simulink model "mpc_cvxgen"  (R2015b)
settings: Solver=VariableStepAuto  StartTime=0.0  StopTime=50  FixedStep=Ts  RelTol=1e-3
InitFcn:
  | mpc_trajectory_data_callback
values from neighbouring files (symbols this model uses):
  Ts = 1    [example_mpc_cycle.m]    (also in init_mpc_test.m = 0.2)
undefined symbols (not defined in the file or in its folder): sCoeffs, sPolyorder, sTimes
undefined symbols (not defined in the file): CVXparameters
settings Model: Creator=Daniel  LastModifiedBy=mgreiff
settings SolverCC: AlgebraicLoopSolver=LineSearch

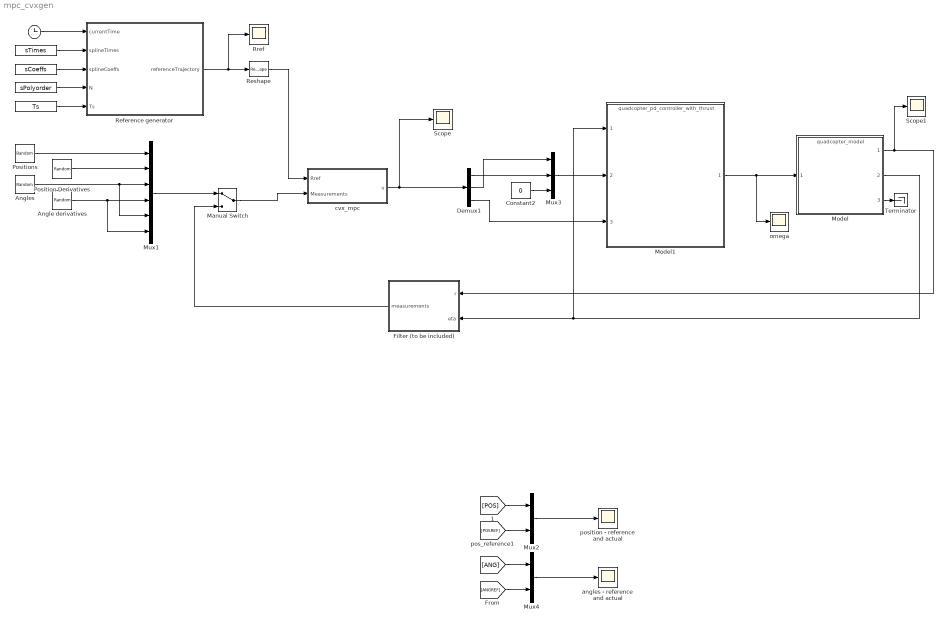
== system mpc_cvxgen ==
  " " : Constant  Value=Ts
  "  " : Constant  Value=sPolyorder
  "   " : Constant  Value=sCoeffs
  "    " : Constant  Value=sTimes
  "      " : Clock
  "  angles - reference and actual" : Scope
  "  position - reference and actual" : Scope
  Angle derivatives : RandomNumber  Variance=0.1  SampleTime=Ts
  Angles : RandomNumber  Variance=0.1  SampleTime=Ts
  Constant2 : Constant  Value=0
  Demux1 : Demux  Outputs=3
  Filter (to be included) : Subsystem
  Manual Switch : ManualSwitch
  Model : ModelReference  ModelNameDialog=quadcopter_model.mdl  SimulationMode=Normal  ModelReferenceVersion=1.114  CopyOfModelName=quadcopter_model.mdl
  Model1 : ModelReference  ModelNameDialog=quadcopter_pd_controller_with_thrust.mdl  SimulationMode=Normal  ModelReferenceVersion=1.70  CopyOfModelName=quadcopter_pd_controller_with_thrust.mdl
  Mux1 : Mux  Inputs=6
  Mux2 : Mux  Inputs=2
  Mux3 : Mux  Inputs=3
  Mux4 : Mux  Inputs=2
  Position Derivatives : RandomNumber  Mean=[0,0,0]  Variance=0.1  SampleTime=Ts
  Positions : RandomNumber  Mean=[0,0,0]  Variance=0.1  SampleTime=Ts
  Reference generator : MATLAB Function  TreatAsAtomicUnit=on
  Reshape : Reshape
  Rref : Scope
  Scope : Scope
  Scope1 : Scope
  Terminator : Terminator
  cvx_mpc : Subsystem  mask{md=CVXparameters}
      mask prompts: md "MPCData"
  "omega " : Scope
  wires:
  Angles/1 -> Mux1/5, Mux1/3
  Angle derivatives/1 -> Mux1/6, Mux1/4
  Positions/1 -> Mux1/1
  Position Derivatives/1 -> Mux1/2
  "      "/1 -> Reference generator/1(currentTime)
  "    "/1 -> Reference generator/2(splineTimes)
  "   "/1 -> Reference generator/3(splineCoeffs)
  "  "/1 -> Reference generator/4(N)
  " "/1 -> Reference generator/5(Ts)
  Reshape/1 -> cvx_mpc/1(Rref)
  Reference generator/1(referenceTrajectory) -> Rref/1, Reshape/1
  Mux1/1 -> Manual Switch/1
  Manual Switch/1 -> cvx_mpc/2(Measurements)
  cvx_mpc/1(u) -> Scope/1, Demux1/1
  Demux1/3 -> Model1/3
  Mux3/1 -> Model1/2
  Constant2/1 -> Mux3/3
  Demux1/2 -> Mux3/1
  Demux1/1 -> Mux3/2
  Model1/1 -> Model/1, "omega "/1
  [POS] -> Mux2/1
  [POSREF] -> Mux2/2
  Mux2/1 -> "  position - reference and actual"/1
  Model/2 -> Filter (to be included)/2(eta), Model1/1
  Filter (to be included)/1(measurements) -> Manual Switch/2
  [ANG] -> Mux4/1
  [ANGREF] -> Mux4/2
  Mux4/1 -> "  angles - reference and actual"/1
  Model/1 -> Scope1/1, Filter (to be included)/1(r)
  Model/3 -> Terminator/1

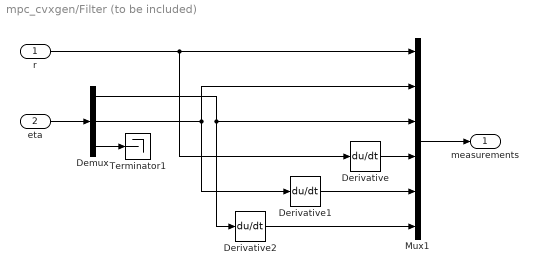
== system mpc_cvxgen/Filter (to be included) ==
  r : Inport
  eta : Inport  Port=2
  Demux : Demux  Outputs=3
  Derivative : Derivative
  Derivative1 : Derivative
  Derivative2 : Derivative
  Mux1 : Mux  Inputs=6
  Terminator1 : Terminator
  measurements : Outport
  wires:
  Demux/1 -> Mux1/3, Derivative2/1
  Derivative/1 -> Mux1/4
  Derivative2/1 -> Mux1/6
  Demux/3 -> Terminator1/1
  Demux/2 -> Mux1/2, Derivative1/1
  Derivative1/1 -> Mux1/5
  r/1 -> Derivative/1, Mux1/1
  eta/1 -> Demux/1
  Mux1/1 -> measurements/1

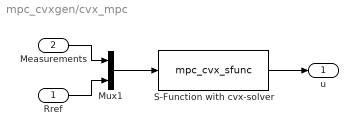
== system mpc_cvxgen/cvx_mpc ==
  Rref : Inport
  Measurements : Inport  Port=2
  Mux1 : Mux  Inputs=2
  S-Function with cvx-solver : S-Function  FunctionName=mpc_cvx_sfunc  Parameters=CVXparameters  SFunctionDeploymentMode=off  EnableBusSupport=off
  u : Outport
  wires:
  Measurements/1 -> Mux1/1
  Rref/1 -> Mux1/2
  S-Function with cvx-solver/1 -> u/1
  Mux1/1 -> S-Function with cvx-solver/1

== matlab function mpc_cvxgen/Reference generator ==
  data: currentTime input; referenceTrajectory output; splineTimes input; splineCoeffs input; N input; Ts input
function referenceTrajectory = fcn(currentTime, splineTimes, splineCoeffs, N, Ts)
%#codegen

predHorizon = 10 + 1; % Number of points on the prediction horizon

times = currentTime + Ts.* (0:predHorizon-1);
referenceTrajectory = zeros(10,predHorizon);

for ii = 1:predHorizon
    % Finds the spline to evaluate
    T = times(ii);
    splineNumber = sum(splineTimes <=  T);

    % Treats the case when the time is outside the defined interval [t_0,t_s]
    if splineNumber == 0
        %disp('Tried to evaluate spline before t_0, setting reference to the initial spline point.')
        T = splineTimes(1);
        splineNumber = 1;
    elseif T >= splineTimes(end)
        %disp('Tried to evaluate spline after t_s, keeping position in terinal spline point')
        T = splineTimes(end);
        splineNumber = length(splineCoeffs(:,1))/(N + 1);
    end
    % Evaluates splines and stores data in referenceTrajectory
    for dim = 1:3
        startIndex = (N + 1) * (splineNumber - 1) + 1;
        endIndex = (N + 1) * splineNumber;
        poscoeff = splineCoeffs(startIndex:endIndex,dim);
        poscoeff = poscoeff(end:-1:1); % Reverses for polyval
        tt = T - splineTimes(splineNumber);

        % Position
        referenceTrajectory(dim,ii) = polyval(poscoeff,tt);

        % Velocity
        poscoeff(end) = [];
        velcoeff = (length(poscoeff):-1:1)'.*poscoeff; 
        referenceTrajectory(dim + 3,ii) = polyval(velcoeff,tt);
    end
end
